simulink model "b01_OSnScheduler"  (R2024a)
settings: Solver=FixedStepDiscrete  StartTime=0.0  StopTime=1  FixedStep=mSim.dTime  MaxStep=Define.sModelSampleTime  RelTol=7.1420e-05
undefined symbols (not defined in the file): B01SCHED
settings Model: Creator=user  LastModifiedBy=admin
settings SolverCC: MaxConsecutiveZCs=10000  ZeroCrossAlgorithm=Adaptive  AlgebraicLoopSolver=TrustRegion
settings DataIOCC: SaveOutput=off  DSMLogging=off  InspectSignalLogs=on  SaveTime=off  SignalLoggingName=logsout_Validator
settings OptimizationCC: BlockReduction=off  DefaultParameterBehavior=Inlined  UseDivisionForNetSlopeComputation=UseDivisionForReciprocalsOfIntegersOnly  GainParamInheritBuiltInType=on  UseFloatMulNetSlope=on  DefaultUnderspecifiedDataType=single  InlineInvariantSignals=on  BitwiseOrLogicalOp=Logical operator  PassReuseOutputArgsAs=Individual arguments  EfficientFloat2IntCast=on  LifeSpan=Inf  OptimizeBlockOrder=speed  DifferentSizesBufferReuse=on  EfficientTunableParamExpr=on
settings DebuggingCC: SignalInfNanChecking=error  SignalRangeChecking=error  ReadBeforeWriteMsg=EnableAllAsError  WriteAfterWriteMsg=EnableAllAsError  WriteAfterReadMsg=EnableAllAsError  AlgebraicLoopMsg=error  ArtificialAlgebraicLoopMsg=error  SaveWithDisabledLinksMsg=error  SaveWithParameterizedLinksMsg=error  BlockPriorityViolationMsg=error  SolverPrmCheckMsg=error  InheritedTsInSrcMsg=error  SingleTaskRateTransMsg=error  TasksWithSamePriorityMsg=error  SigSpecEnsureSampleTimeMsg=error  CheckMatrixSingularityMsg=error  IntegerOverflowMsg=error  ParameterUnderflowMsg=error  ParameterPrecisionLossMsg=error  ParameterTunabilityLossMsg=error  UnderSpecifiedDataTypeMsg=error  UnnecessaryDatatypeConvMsg=warning  VectorMatrixConversionMsg=error  SignalLabelMismatchMsg=error  UnconnectedInputMsg=error  UnconnectedOutputMsg=error  UnconnectedLineMsg=error  SFcnCompatibilityMsg=error  UniqueDataStoreMsg=error  BusObjectLabelMismatch=error  RootOutportRequireBusObject=error  AssertControl=DisableAll  ModelReferenceIOMismatchMessage=error  UnknownTsInhSupMsg=error  ModelReferenceDataLoggingMessage=error  ModelReferenceSymbolNameMessage=none  StateNameClashWarn=warning  StrictBusMsg=ErrorOnBusTreatedAsVector  NonBusSignalsTreatedAsBus=error  SFInvalidInputDataAccessInChartInitDiag=error  SFTransitionOutsideNaturalParentDiag=error  SFUnreachableExecutionPathDiag=error  SFUndirectedBroadcastEventsDiag=error  SFTransitionActionBeforeConditionDiag=error  SFTemporalDelaySmallerThanSampleTimeDiag=error  SFSelfTransitionDiag=error  SFExecutionAtInitializationDiag=error  IntegerSaturationMsg=error  UnitsInconsistencyMsg=none  VariantConditionMismatch=error
settings HardwareCC: ProdBitPerChar=16  ProdBitPerInt=16  ProdBitPerPointer=32  ProdBitPerSizeT=32  ProdBitPerPtrDiffT=32  ProdLargestAtomicInteger=Integer  ProdLargestAtomicFloat=None  ProdWordSize=16  ProdHWDeviceType=Texas Instruments->C2000
settings ModelReferenceCC: EnableRefExpFcnMdlSchedulingChecks=on  ModelReferenceNumInstancesAllowed=Single
settings SFSimCC: SimUseLocalCustomCode=off  CompileTimeRecursionLimit=0  EnableRuntimeRecursion=off  MATLABDynamicMemAlloc=off  CustomCodeUndefinedFunction=UseInterfaceOnly
settings RTWCC: Description=Embedded Coder  SystemTargetFile=ert.tlc  GenCodeOnly=on  TemplateMakefile=ert_default_tmf  GenerateReport=on  RTWUseLocalCustomCode=off  BuildConfiguration=Faster Runs  IncludeHyperlinkInReport=on  LaunchReport=on  GenerateTraceInfo=on  GenerateTraceReport=on  GenerateTraceReportSl=on  GenerateTraceReportSf=on  GenerateWebview=on  GenerateCodeMetricsReport=on  GenerateCodeReplacementReport=on  GPUComputeCapability=3.5  DLArmComputeVersion=19.05
settings RTWCC: CustomHeaderCode=|
  | #include "Define_Header.h"
  | #include "M1_Interrupt.h"
  | #include "M2_Interrupt.h"
  | #include "Define_DAC.h"
settings CodeAppCC: ForceParamTrailComments=on  IgnoreCustomStorageClasses=off  MATLABFcnDesc=on  MangleLength=4  CustomSymbolStrGlobalVar=GvB01$N$M  CustomSymbolStrType=StrB01$N$M  CustomSymbolStrFcn=$N$M$F  CustomSymbolStrMacro=$N$M  DefineNamingRule=UpperCase  ParamNamingRule=UpperCase  SimulinkBlockComments=off  MATLABSourceComments=on  EnableCustomComments=on  ReqsInCode=on
settings ERTTargetCC: TargetLangStandard=C99 (ISO)  UtilityFuncGeneration=Shared location  MultiwordLength=2048  IncludeMdlTerminateFcn=off  CombineSignalStateStructs=on  SuppressErrorStatus=on  SupportAbsoluteTime=off  SupportNonFinite=off  ParenthesesLevel=Maximum  CastingMode=Standards  GenerateSharedConstants=off  InlinedParameterPlacement=NonHierarchical  ERTSrcFileBannerTemplate=t_code_template.cgt  ERTHdrFileBannerTemplate=t_code_template.cgt  ERTDataSrcFileTemplate=t_code_template.cgt  ERTDataHdrFileTemplate=t_code_template.cgt  ERTCustomFileTemplate=example_file_process.tlc  ERTFilePackagingFormat=CompactWithDataFile  PreserveExpressionOrder=on  SuppressUnreachableDefaultCases=off  EnableSignedLeftShifts=off  EnableSignedRightShifts=off  IndentStyle=Allman  IndentSize=4
settings ConfigComp: CovSaveName=coveragedata  CovMetricSettings=we  CovEnableCumulative=off  CovSaveCumulativeToWorkspaceVar=on  CovSaveSingleToWorkspaceVar=on  CovOutputDir=sldv_output/$ModelName$\sldv_covoutput  PSVerificationMode=BugFinder  PSModelRefIgnoreList=[]  PSEnableModelRefIgnoreList=off  PSModelRefMinMaxVerif=CheckAndConstrain  PSAutoStubLUT=on  DVModelCoverageObjectives=MCDC  DVTestSuiteOptimization=CombinedObjectives (Nonlinear Extended)  DVRebuildModelRepresentation=Always
settings SimscapeCC: SimscapeNormalizeSystem=off

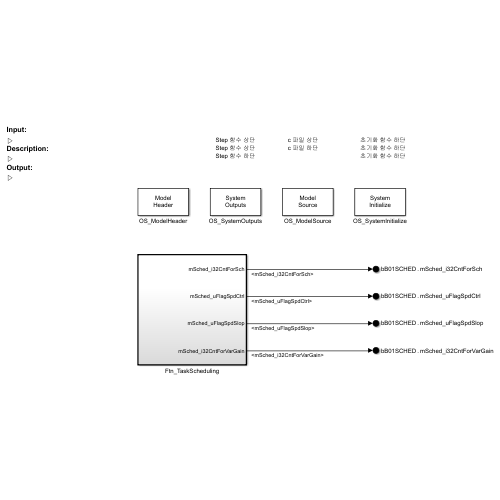
[thumbnail: Simulink's stored preview of the top-level diagram]
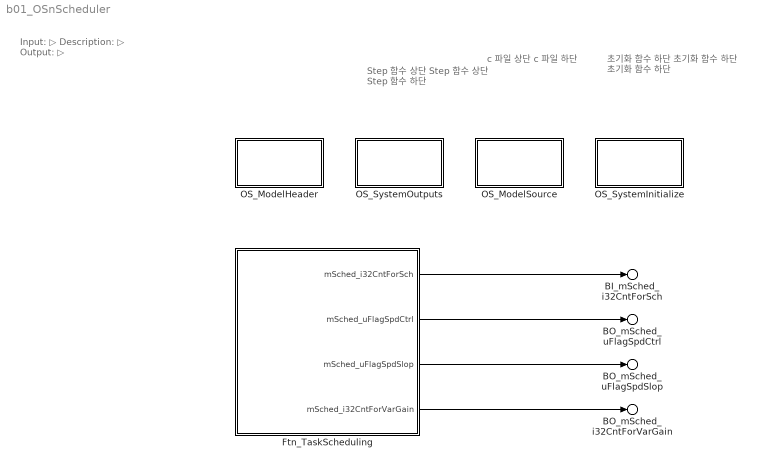
== system b01_OSnScheduler ==
  note: Input:
      | ▷
      | Description:
      | ▷
      | Output:
      | ▷
  note: 초기화 함수 하단
      | 초기화 함수 하단
      | 초기화 함수 하단
  note: c 파일 상단
      | c 파일 하단
  note: Step 함수 상단
      | Step 함수 상단
      | Step 함수 하단
  Ftn_TaskScheduling : Subsystem  Tag=Ftn_CntOuterLoopSENS  TreatAsAtomicUnit=on
      settings: RTWSystemCode=Nonreusable function  RTWFcnNameOpts=Use subsystem name
  OS_ModelHeader : Subsystem  mask(Model Header){ShowInLibBrowser=0}
      mask prompts: ShowInLibBrowser "Simulink:masks:CustCodeMaskParam1_MP"
      settings: CopyFcn=cccopyfcn(gcb)  OpenFcn=ccopenfcn('Model Header')
      mask Help: eval('feval(''rtwprivate'',''rtwhelpview'',''rtw_model_header_block'')');
      mask DialogControl ShowInLibBrowser Prompt: 마스크 파라미터 1:
      mask Display: disp('Model\nHeader');
  OS_ModelSource : Subsystem  mask(Model Source){ShowInLibBrowser=0}
      mask prompts: ShowInLibBrowser "Simulink:masks:CustCodeMaskParam1_MP"
      settings: CopyFcn=cccopyfcn(gcb)  OpenFcn=ccopenfcn('Model Source')
      mask Help: eval('feval(''rtwprivate'',''rtwhelpview'',''rtw_model_source_block'')');
      mask DialogControl ShowInLibBrowser Prompt: 마스크 파라미터 1:
      mask Display: disp('Model\nSource');
  OS_SystemInitialize : Subsystem  mask(System Initialize){ShowInLibBrowser=0}
      mask prompts: ShowInLibBrowser "Simulink:masks:CustCodeMaskParam1_MP"
      settings: CopyFcn=cccopyfcn(gcb)  OpenFcn=ccopenfcn('System Initialize Function')
      mask Help: eval('feval(''rtwprivate'',''rtwhelpview'',''rtw_sys_initialize_block'')');
      mask DialogControl ShowInLibBrowser Prompt: 마스크 파라미터 1:
      mask Display: disp('System\nInitialize');
  OS_SystemOutputs : Subsystem  mask(System Outputs){ShowInLibBrowser=0}
      mask prompts: ShowInLibBrowser "Simulink:masks:CustCodeMaskParam1_MP"
      settings: CopyFcn=cccopyfcn(gcb)  OpenFcn=ccopenfcn('System Outputs Function')
      mask Help: eval('feval(''rtwprivate'',''rtwhelpview'',''rtw_sys_outputs_block'')');
      mask DialogControl ShowInLibBrowser Prompt: 마스크 파라미터 1:
      mask Display: disp('System\nOutputs');
  BO_mSched_uFlagSpdCtrl : Outport  Description=■ 설명: Speed Control 스케쥴 카운터  PortName=bB01SCHED  Element=mSched_uFlagSpdCtrl
  BO_mSched_uFlagSpdSlop : Outport  Description=■ 설명: 속도 지령 Slop 스케쥴 카운터  PortName=bB01SCHED  Element=mSched_uFlagSpdSlop
  BI_mSched_i32CntForSch : Outport  Description=■ 설명: 메인 스케쥴 카운터  PortName=bB01SCHED  Element=mSched_i32CntForSch
  BO_mSched_i32CntForVarGain : Outport  Description=■ 설명: 가변게인 스케쥴 카운터  PortName=bB01SCHED  Element=mSched_i32CntForVarGain
  wires:
  Ftn_TaskScheduling/3(mSched_uFlagSpdSlop) -> BO_mSched_uFlagSpdSlop/1
  Ftn_TaskScheduling/1(mSched_i32CntForSch) -> BI_mSched_i32CntForSch/1
  Ftn_TaskScheduling/2(mSched_uFlagSpdCtrl) -> BO_mSched_uFlagSpdCtrl/1
  Ftn_TaskScheduling/4(mSched_i32CntForVarGain) -> BO_mSched_i32CntForVarGain/1

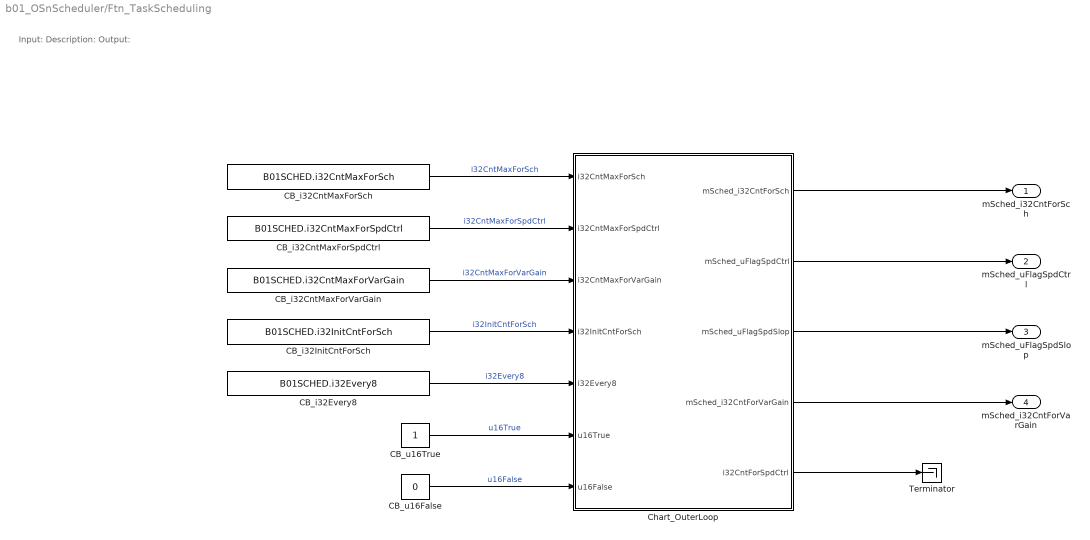
== system b01_OSnScheduler/Ftn_TaskScheduling ==
  note: Input:
      | Description:
      | Output:
  CB_i32CntMaxForSch : Constant  Value=B01SCHED.i32CntMaxForSch
  CB_i32CntMaxForSpdCtrl : Constant  Value=B01SCHED.i32CntMaxForSpdCtrl
  CB_i32CntMaxForVarGain : Constant  Value=B01SCHED.i32CntMaxForVarGain
  CB_i32Every8 : Constant  Value=B01SCHED.i32Every8
  CB_i32InitCntForSch : Constant  Value=B01SCHED.i32InitCntForSch
  CB_u16False : Constant  Value=0  OutDataTypeStr=uint16
  CB_u16True : Constant  OutDataTypeStr=uint16
  Chart_OuterLoop : Stateflow chart  TreatAsAtomicUnit=on
  Terminator : Terminator
  mSched_i32CntForSch : Outport  Description=■ 설명: 메인 스케쥴 카운터  OutMin=0  OutMax=50  VectorParamsAs1DForOutWhenUnconnected=off
  mSched_uFlagSpdCtrl : Outport  Description=■ 설명: Speed Control 스케쥴 카운터  Port=2  OutMin=0  OutMax=1
  mSched_uFlagSpdSlop : Outport  Description=■ 설명: 속도 지령 Slop 스케쥴 카운터  Port=3  OutMin=0  OutMax=1
  mSched_i32CntForVarGain : Outport  Description=■ 설명: 가변게인 스케쥴 카운터  Port=4  OutMin=0  OutMax=3
  wires:
  CB_i32CntMaxForSch/1 -> Chart_OuterLoop/1(i32CntMaxForSch)  "i32CntMaxForSch"
  Chart_OuterLoop/1(mSched_i32CntForSch) -> mSched_i32CntForSch/1
  CB_u16True/1 -> Chart_OuterLoop/6(u16True)  "u16True"
  CB_u16False/1 -> Chart_OuterLoop/7(u16False)  "u16False"
  CB_i32CntMaxForSpdCtrl/1 -> Chart_OuterLoop/2(i32CntMaxForSpdCtrl)  "i32CntMaxForSpdCtrl"
  Chart_OuterLoop/5(i32CntForSpdCtrl) -> Terminator/1
  Chart_OuterLoop/3(mSched_uFlagSpdSlop) -> mSched_uFlagSpdSlop/1
  Chart_OuterLoop/2(mSched_uFlagSpdCtrl) -> mSched_uFlagSpdCtrl/1
  CB_i32CntMaxForVarGain/1 -> Chart_OuterLoop/3(i32CntMaxForVarGain)  "i32CntMaxForVarGain"
  Chart_OuterLoop/4(mSched_i32CntForVarGain) -> mSched_i32CntForVarGain/1
  CB_i32Every8/1 -> Chart_OuterLoop/5(i32Every8)  "i32Every8"
  CB_i32InitCntForSch/1 -> Chart_OuterLoop/4(i32InitCntForSch)  "i32InitCntForSch"

== system b01_OSnScheduler/OS_ModelHeader ==

== system b01_OSnScheduler/OS_ModelSource ==

== system b01_OSnScheduler/OS_SystemInitialize ==

== system b01_OSnScheduler/OS_SystemOutputs ==

== stateflow chart b01_OSnScheduler/Ftn_TaskScheduling/Chart_OuterLoop ==
  (default) -> (junction 2)
  (junction 2) -> (junction 3) [order 1] : [mSched_i32CntForSch >= i32CntMaxForSch]
  (junction 2) -> (junction 13) [order 2] : {
      | mSched_i32CntForSch = mSched_i32CntForSch + i32InitCntForSch;
      | }
  (junction 3) -> (junction 4) : {
      | mSched_i32CntForSch = i32InitCntForSch;
      | i32CntForSpdCtrl = i32InitCntForSch;
      | }
  (junction 4) -> (junction 13)
  (junction 13) -> (junction 34)
  (junction 34) -> (junction 38) [order 1] : [i32CntForSpdCtrl >= i32CntMaxForSpdCtrl]
  (junction 34) -> (junction 46) [order 2] : {
      | i32CntForSpdCtrl = i32CntForSpdCtrl + i32InitCntForSch;
      | mSched_uFlagSpdCtrl = u16False;
      | }
  (junction 38) -> (junction 39) : {
      | i32CntForSpdCtrl = i32InitCntForSch;
      | mSched_uFlagSpdCtrl = u16True;
      | }
  (junction 46) -> (junction 48) [order 1] : [i32CntForSpdCtrl == i32Every8]
  (junction 46) -> (junction 36) [order 2] : {
      | mSched_uFlagSpdSlop = u16False;
      | }
  (junction 48) -> (junction 49) : {
      | mSched_uFlagSpdSlop = u16True;
      | }
  (junction 49) -> (junction 36)
  (junction 39) -> (junction 49)
  (junction 36) -> (junction 79)
  (junction 79) -> (junction 78) [order 1] : [mSched_i32CntForVarGain >= i32CntMaxForVarGain]
  (junction 79) -> (junction 80) [order 2] : {
      | mSched_i32CntForVarGain = mSched_i32CntForVarGain + i32InitCntForSch;
      | }
  (junction 78) -> (junction 83) : {
      | mSched_i32CntForVarGain = i32InitCntForSch;
      | }
  (junction 83) -> (junction 80)
  (junction 80) -> (junction 82)
  data: mSched_i32CntForSch output int32; i32CntMaxForSch input int32; i32CntMaxForSpdCtrl input; i32CntMaxForVarGain input; i32InitCntForSch input =1; i32Every8 input int32 =8; u16True input; u16False input; mSched_uFlagSpdCtrl output uint16; mSched_uFlagSpdSlop output uint16; mSched_i32CntForVarGain output int32; i32CntForSpdCtrl output int32 =1
